simulink model "Model_SD_CIFB_k2"  (R2023a)
settings: Solver=VariableStepAuto  StartTime=0.0  StopTime=Tstop  RelTol=1e-3  EnableMultiTasking=on
values from neighbouring files (symbols this model uses):
  Amp = 10^(Av/20)*FS    (= 0.501187233627)    [run_Model_SD_CIFB_k2.m]
  fs = 2*BA*OSR    (= 2560000)    [run_Model_SD_CIFB_k2.m]
  k = 10^(gain/20)    (= 10000)    [run_Model_SD_CIFB_k2.m]
  OSR = 64    [run_Model_SD_CIFB_k2.m]
  ts = 1/fs    (= 3.90625e-07)    [run_Model_SD_CIFB_k2.m]
  w0 = GBW/k    (= 5000)    [run_Model_SD_CIFB_k2.m]
  win = 2*pi*fin    [run_Model_SD_CIFB_k2.m]
settings Model: Creator=cellierr  LastModifiedBy=Dorian
settings SolverCC: AlgebraicLoopSolver=TrustRegion
settings DataIOCC: LimitDataPoints=on  SaveFormat=Array  SignalLoggingSaveFormat=ModelDataLogs  ReturnWorkspaceOutputs=off
settings OptimizationCC: ExpressionDepthLimit=2147483647  InitFltsAndDblsToZero=on  LifeSpan=inf
settings DebuggingCC: SaveWithParameterizedLinksMsg=none  UnderspecifiedInitializationDetection=Classic  MergeDetectMultiDrivingBlocksExec=none  SolverPrmCheckMsg=warning  FcnCallInpInsideContextMsg=warning  UnconnectedInputMsg=warning  UnconnectedOutputMsg=warning  UnconnectedLineMsg=warning  StateNameClashWarn=warning  SFUnexpectedBacktrackingDiag=warning  SFNoUnconditionalDefaultTransitionDiag=warning  SFExecutionAtInitializationDiag=none  ArithmeticOperatorsInVariantConditions=warning
settings HardwareCC: ProdBitPerPointer=32  ProdBitPerSizeT=32  ProdBitPerPtrDiffT=32  ProdLargestAtomicFloat=None  ProdIntDivRoundTo=Undefined  ProdEndianess=Unspecified  ProdWordSize=32  ProdHWDeviceType=32-bit Generic
settings ModelReferenceCC: EnableRefExpFcnMdlSchedulingChecks=on  PropagateSignalLabelsOutOfModel=off
settings SFSimCC: SimUseLocalCustomCode=off  CustomCodeUndefinedFunction=UseInterfaceOnly
settings RTWCC: RTWUseLocalCustomCode=off
settings CodeAppCC: StateflowObjectComments=on
settings GRTTargetCC: TargetFcnLib=ansi_tfl_tmw.mat  TargetLangStandard=C89/C90 (ANSI)  CombineOutputUpdateFcns=off  GRTInterface=on
settings ConfigComp: CovMetricSettings=dw  CovSaveCumulativeToWorkspaceVar=on  CovSaveSingleToWorkspaceVar=on  CovExternalEMLEnable=off  CovSFcnEnable=off

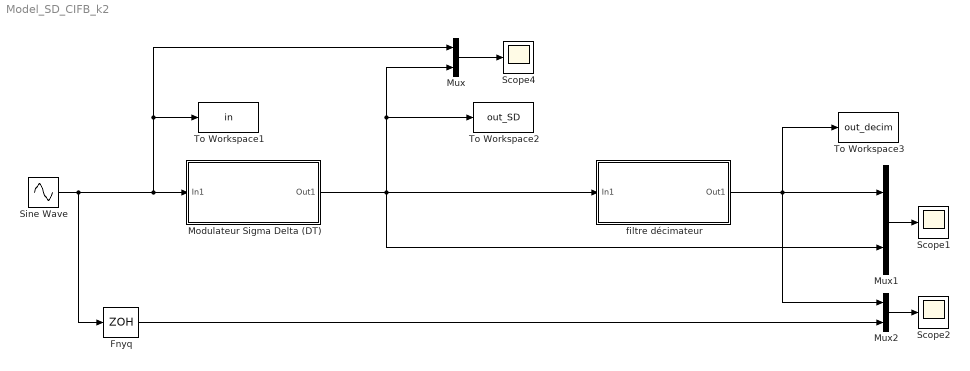
== system Model_SD_CIFB_k2 ==
  Fnyq : ZeroOrderHold  SampleTime=ts*OSR
  Modulateur Sigma Delta (DT) : Subsystem
  Mux : Mux  Inputs=2
  Mux1 : Mux  Inputs=2
  Mux2 : Mux  Inputs=2
  Scope1 : Scope
  Scope2 : Scope
  Scope4 : Scope
  Sine Wave : Sin  Amplitude=Amp  Frequency=win  SampleTime=0
  To Workspace1 : ToWorkspace  VariableName=in  SampleTime=-1
  To Workspace2 : ToWorkspace  VariableName=out_SD  SampleTime=-1
  To Workspace3 : ToWorkspace  VariableName=out_decim  SampleTime=ts
  filtre décimateur : Subsystem
  wires:
  Sine Wave/1 -> Modulateur Sigma Delta (DT)/1(In1), Mux/1, To Workspace1/1, Fnyq/1
  Mux/1 -> Scope4/1
  Mux1/1 -> Scope1/1
  Fnyq/1 -> Mux2/2
  Mux2/1 -> Scope2/1
  Modulateur Sigma Delta (DT)/1(Out1) -> Mux1/2, filtre décimateur/1(In1), To Workspace2/1, Mux/2
  filtre décimateur/1(Out1) -> Mux2/1, To Workspace3/1, Mux1/1

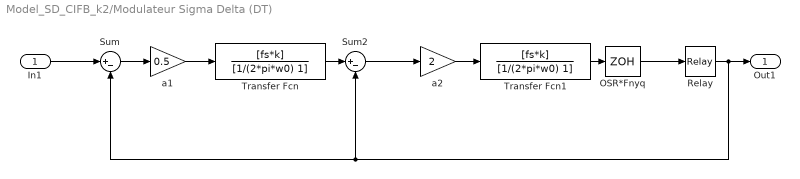
== system Model_SD_CIFB_k2/Modulateur Sigma Delta (DT) ==
  In1 : Inport
  OSR*Fnyq : ZeroOrderHold  SampleTime=1/(fs)
  Relay : Relay  OnSwitchValue=0  OffSwitchValue=0  OffOutputValue=-1
  Sum : Sum  Inputs=|+-
  Sum2 : Sum  Inputs=|+-
  Transfer Fcn : TransferFcn  Numerator=[fs*k]  Denominator=[1/(2*pi*w0) 1]
  Transfer Fcn1 : TransferFcn  Numerator=[fs*k]  Denominator=[1/(2*pi*w0) 1]
  a1 : Gain  Gain=0.5
  a2 : Gain  Gain=2
  Out1 : Outport
  wires:
  In1/1 -> Sum/1
  Sum/1 -> a1/1
  a1/1 -> Transfer Fcn/1
  Sum2/1 -> a2/1
  Relay/1 -> Sum2/2, Sum/2, Out1/1
  Transfer Fcn/1 -> Sum2/1
  a2/1 -> Transfer Fcn1/1
  Transfer Fcn1/1 -> OSR*Fnyq/1
  OSR*Fnyq/1 -> Relay/1

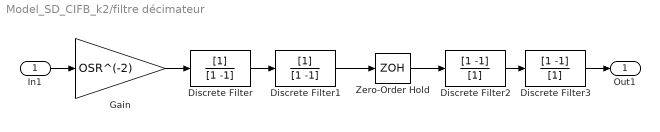
== system Model_SD_CIFB_k2/filtre décimateur ==
  In1 : Inport
  Discrete Filter : DiscreteFilter  Denominator=[1 -1]
  Discrete Filter1 : DiscreteFilter  Denominator=[1 -1]
  Discrete Filter2 : DiscreteFilter  Numerator=[1 -1]  Denominator=[1]  SampleTime=ts*OSR
  Discrete Filter3 : DiscreteFilter  Numerator=[1 -1]  Denominator=[1]  SampleTime=ts*OSR
  Gain : Gain  Gain=OSR^(-2)  SaturateOnIntegerOverflow=on  OutDataTypeStr=Inherit: Same as input  ParamDataTypeStr=Inherit: Same as input
  Zero-Order Hold : ZeroOrderHold  SampleTime=ts*OSR
  Out1 : Outport
  wires:
  In1/1 -> Gain/1
  Discrete Filter3/1 -> Out1/1
  Gain/1 -> Discrete Filter/1
  Discrete Filter/1 -> Discrete Filter1/1
  Discrete Filter2/1 -> Discrete Filter3/1
  Discrete Filter1/1 -> Zero-Order Hold/1
  Zero-Order Hold/1 -> Discrete Filter2/1
